simulink model "feedbackLineariz"  (Simulink 8.0)
settings: Solver=FixedStepDiscrete  StartTime=0.0  StopTime=inf  FixedStep=Ts  RelTol=1e-3
InitFcn:
  | initFeedLin;
values from neighbouring files (symbols this model uses):
  kp = diag([30*ones(1,3),7*ones(1,22)])    [initFeedLin.m]
libraries: WBCLibrary x11, utility x1
settings Model: Creator=iron  LastModifiedBy=daniele
settings DataIOCC: SignalLoggingSaveFormat=ModelDataLogs
settings DebuggingCC: FcnCallInpInsideContextMsg=UseLocalSettings
settings GRTTargetCC: CombineOutputUpdateFcns=off  GRTInterface=on

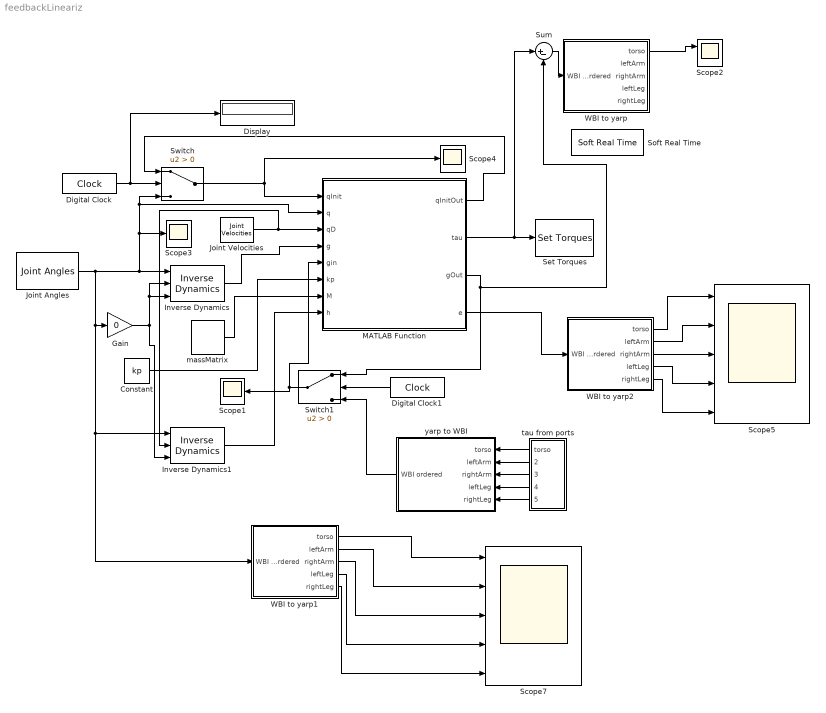
== system feedbackLineariz ==
  Constant : Constant  Value=kp
  Digital Clock : DigitalClock  SampleTime=-1
  Digital Clock1 : DigitalClock  SampleTime=-1
  Display : Display
  Gain : Gain  Gain=0
  Inverse Dynamics : WBCLibrary/wholeBodyModel/Dynamics/Inverse Dynamics  robotName=robotName  localName=localName
  Inverse Dynamics1 : WBCLibrary/wholeBodyModel/Dynamics/Inverse Dynamics  robotName=robotName  localName=localName
  Joint Angles : WBCLibrary/wholeBodyStates/Joint Angles  robotName=robotName  localName=localName
  Joint Velocities : WBCLibrary/wholeBodyStates/Joint Velocities  robotName=robotName  localName=localName
  MATLAB Function : MATLAB Function  TreatAsAtomicUnit=on
  Scope1 : Scope
      settings: YMin=-0.6  YMax=0.8
  Scope2 : Scope  NumInputPorts=2
      settings: YMin=-7~-5  YMax=6~5
  Scope3 : Scope
      settings: YMin=-0.6  YMax=0.8  SaveName=ScopeData3
  Scope4 : Scope
      settings: YMin=-0.6  YMax=0.8  SaveName=ScopeData4
  Scope5 : Scope  NumInputPorts=5
      settings: TimeRange=4.5  YMin=-0.1~-0.1~-0.2~-0.1~-0.1  YMax=0.3~0.3~0.2~0.3~0.3  SaveName=ScopeData2
  Scope7 : Scope  NumInputPorts=5
      settings: YMin=-0.5~-5~-5~-5~-5  YMax=4.75~5~5~5~5  SaveName=ScopeData6
  Set Torques : WBCLibrary/wholeBodyActuators/Set Torques  val=6  robotName=robotName  localName=localName
  Soft Real Time : utility/Soft Real Time  x=Ts
  Sum : Sum  Inputs=|+-
  Switch : Switch  Criteria=u2 > Threshold
  Switch1 : Switch  Criteria=u2 > Threshold
  WBI to yarp : Subsystem
  WBI to yarp1 : Subsystem
  WBI to yarp2 : Subsystem
  massMatrix : WBCLibrary/wholeBodyModel/Dynamics/massMatrix  val=8  robotname=robotName  localname=localName
  tau from ports : Subsystem
  yarp to WBI : Subsystem
  wires:
  Joint Angles/1 -> Inverse Dynamics1/1, WBI to yarp1/1(WBI ordered), Gain/1, Scope3/1, MATLAB Function/2(q), Switch/3, Inverse Dynamics/1
  Gain/1 -> Inverse Dynamics/2, Inverse Dynamics/3, Inverse Dynamics1/3
  Digital Clock/1 -> Display/1, Switch/2
  Switch/1 -> Scope4/1, MATLAB Function/1(qInit)
  MATLAB Function/1(qInitOut) -> Switch/1
  Joint Velocities/1 -> Inverse Dynamics1/2, MATLAB Function/3(qD)
  MATLAB Function/2(tau) -> Sum/1, Set Torques/1
  Digital Clock1/1 -> Switch1/2
  tau from ports/1(torso) -> yarp to WBI/1(torso)
  tau from ports/2(leftArm) -> yarp to WBI/2(leftArm)
  tau from ports/3(rightArm) -> yarp to WBI/3(rightArm)
  tau from ports/4(leftLeg) -> yarp to WBI/4(leftLeg)
  tau from ports/5(rightLeg) -> yarp to WBI/5(rightLeg)
  Switch1/1 -> Scope1/1, MATLAB Function/5(gin)
  MATLAB Function/3(gOut) -> Sum/2, Switch1/1
  yarp to WBI/1(WBI ordered) -> Switch1/3
  Constant/1 -> MATLAB Function/6(kp)
  Inverse Dynamics/1 -> MATLAB Function/4(g)
  massMatrix/1 -> MATLAB Function/7(M)
  Inverse Dynamics1/1 -> MATLAB Function/8(h)
  WBI to yarp/1(torso) -> Scope2/1
  Sum/1 -> WBI to yarp/1(WBI ordered)
  WBI to yarp1/1(torso) -> Scope7/1
  WBI to yarp1/2(leftArm) -> Scope7/2
  WBI to yarp1/3(rightArm) -> Scope7/3
  WBI to yarp1/4(leftLeg) -> Scope7/4
  WBI to yarp1/5(rightLeg) -> Scope7/5
  WBI to yarp2/2(leftArm) -> Scope5/2
  WBI to yarp2/1(torso) -> Scope5/1
  WBI to yarp2/3(rightArm) -> Scope5/3
  WBI to yarp2/4(leftLeg) -> Scope5/4
  WBI to yarp2/5(rightLeg) -> Scope5/5
  MATLAB Function/4(e) -> WBI to yarp2/1(WBI ordered)

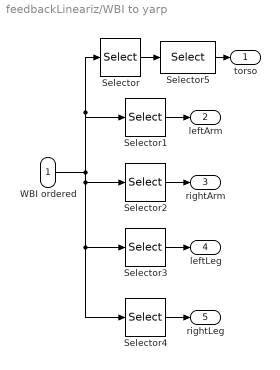
== system feedbackLineariz/WBI to yarp ==
  WBI ordered : Inport
  Selector : Selector  InputPortWidth=25  IndexOptions=Index vector (dialog)  Indices=[1 2 3]  OutputSizes=1
  Selector1 : Selector  InputPortWidth=25  IndexOptions=Index vector (dialog)  Indices=[4 5 6 7 8]  OutputSizes=1
  Selector2 : Selector  InputPortWidth=25  IndexOptions=Index vector (dialog)  Indices=[9 10 11 12 13]  OutputSizes=1
  Selector3 : Selector  InputPortWidth=25  IndexOptions=Index vector (dialog)  Indices=[14 15 16 17 18 19]  OutputSizes=1
  Selector4 : Selector  InputPortWidth=25  IndexOptions=Index vector (dialog)  Indices=[20 21 22 23 24 25]  OutputSizes=1
  Selector5 : Selector  InputPortWidth=3  IndexOptions=Index vector (dialog)  Indices=[3 2 1]  OutputSizes=1
  torso : Outport
  leftArm : Outport  Port=2
  rightArm : Outport  Port=3
  leftLeg : Outport  Port=4
  rightLeg : Outport  Port=5
  wires:
  Selector1/1 -> leftArm/1
  Selector2/1 -> rightArm/1
  Selector3/1 -> leftLeg/1
  Selector4/1 -> rightLeg/1
  WBI ordered/1 -> Selector/1, Selector1/1, Selector2/1, Selector4/1, Selector3/1
  Selector/1 -> Selector5/1
  Selector5/1 -> torso/1

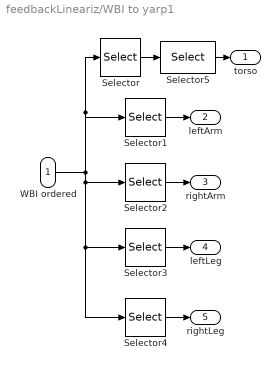
== system feedbackLineariz/WBI to yarp1 ==
  WBI ordered : Inport
  Selector : Selector  InputPortWidth=25  IndexOptions=Index vector (dialog)  Indices=[1 2 3]  OutputSizes=1
  Selector1 : Selector  InputPortWidth=25  IndexOptions=Index vector (dialog)  Indices=[4 5 6 7 8]  OutputSizes=1
  Selector2 : Selector  InputPortWidth=25  IndexOptions=Index vector (dialog)  Indices=[9 10 11 12 13]  OutputSizes=1
  Selector3 : Selector  InputPortWidth=25  IndexOptions=Index vector (dialog)  Indices=[14 15 16 17 18 19]  OutputSizes=1
  Selector4 : Selector  InputPortWidth=25  IndexOptions=Index vector (dialog)  Indices=[20 21 22 23 24 25]  OutputSizes=1
  Selector5 : Selector  InputPortWidth=3  IndexOptions=Index vector (dialog)  Indices=[3 2 1]  OutputSizes=1
  torso : Outport
  leftArm : Outport  Port=2
  rightArm : Outport  Port=3
  leftLeg : Outport  Port=4
  rightLeg : Outport  Port=5
  wires:
  Selector1/1 -> leftArm/1
  Selector2/1 -> rightArm/1
  Selector3/1 -> leftLeg/1
  Selector4/1 -> rightLeg/1
  WBI ordered/1 -> Selector/1, Selector1/1, Selector2/1, Selector4/1, Selector3/1
  Selector/1 -> Selector5/1
  Selector5/1 -> torso/1

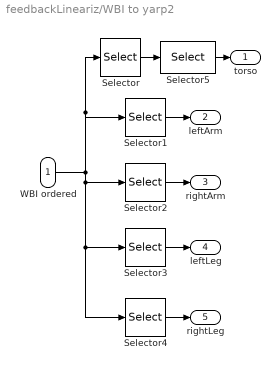
== system feedbackLineariz/WBI to yarp2 ==
  WBI ordered : Inport
  Selector : Selector  InputPortWidth=25  IndexOptions=Index vector (dialog)  Indices=[1 2 3]  OutputSizes=1
  Selector1 : Selector  InputPortWidth=25  IndexOptions=Index vector (dialog)  Indices=[4 5 6 7 8]  OutputSizes=1
  Selector2 : Selector  InputPortWidth=25  IndexOptions=Index vector (dialog)  Indices=[9 10 11 12 13]  OutputSizes=1
  Selector3 : Selector  InputPortWidth=25  IndexOptions=Index vector (dialog)  Indices=[14 15 16 17 18 19]  OutputSizes=1
  Selector4 : Selector  InputPortWidth=25  IndexOptions=Index vector (dialog)  Indices=[20 21 22 23 24 25]  OutputSizes=1
  Selector5 : Selector  InputPortWidth=3  IndexOptions=Index vector (dialog)  Indices=[3 2 1]  OutputSizes=1
  torso : Outport
  leftArm : Outport  Port=2
  rightArm : Outport  Port=3
  leftLeg : Outport  Port=4
  rightLeg : Outport  Port=5
  wires:
  Selector1/1 -> leftArm/1
  Selector2/1 -> rightArm/1
  Selector3/1 -> leftLeg/1
  Selector4/1 -> rightLeg/1
  WBI ordered/1 -> Selector/1, Selector1/1, Selector2/1, Selector4/1, Selector3/1
  Selector/1 -> Selector5/1
  Selector5/1 -> torso/1

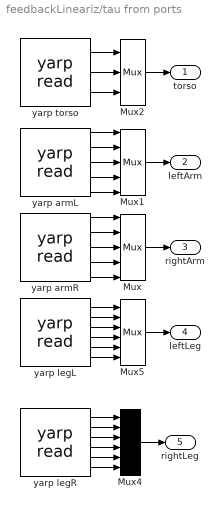
== system feedbackLineariz/tau from ports ==
  Mux : Mux  Inputs=5
  Mux1 : Mux  Inputs=5
  Mux2 : Mux  Inputs=3
  Mux4 : Mux  Inputs=6
  Mux5 : Mux  Inputs=6
  yarp armL : WBCLibrary/Utilities/yarp read  from='/icubGazeboSim/left_arm/analog:o/torques'  to='/tmp2:i'  num=5
  yarp armR : WBCLibrary/Utilities/yarp read  from='/icubGazeboSim/right_arm/analog:o/torques'  to='/tmp3:i'  num=5
  yarp legL : WBCLibrary/Utilities/yarp read  from='/icubGazeboSim/left_leg/analog:o/torques'  to='/tmp4:i'  num=6
  yarp legR : WBCLibrary/Utilities/yarp read  from='/icubGazeboSim/right_leg/analog:o/torques'  to='/tmp5:i'  num=6
  yarp torso : WBCLibrary/Utilities/yarp read  from='/icubGazeboSim/torso/analog:o/torques'  to='/tmp1:i'  num=3
  torso : Outport
  leftArm : Outport  Port=2
  rightArm : Outport  Port=3
  leftLeg : Outport  Port=4
  rightLeg : Outport  Port=5
  wires:
  yarp armR/1 -> Mux/1
  yarp armR/2 -> Mux/2
  yarp armR/3 -> Mux/3
  yarp armR/4 -> Mux/4
  yarp armR/5 -> Mux/5
  yarp armL/1 -> Mux1/1
  yarp armL/2 -> Mux1/2
  yarp armL/3 -> Mux1/3
  yarp armL/4 -> Mux1/4
  yarp armL/5 -> Mux1/5
  yarp torso/1 -> Mux2/1
  yarp torso/2 -> Mux2/2
  yarp torso/3 -> Mux2/3
  yarp legL/1 -> Mux5/1
  yarp legL/2 -> Mux5/2
  yarp legL/3 -> Mux5/3
  yarp legL/4 -> Mux5/4
  yarp legL/5 -> Mux5/5
  yarp legL/6 -> Mux5/6
  yarp legR/1 -> Mux4/1
  yarp legR/2 -> Mux4/2
  yarp legR/3 -> Mux4/3
  yarp legR/4 -> Mux4/4
  yarp legR/5 -> Mux4/5
  yarp legR/6 -> Mux4/6
  Mux2/1 -> torso/1
  Mux1/1 -> leftArm/1
  Mux/1 -> rightArm/1
  Mux5/1 -> leftLeg/1
  Mux4/1 -> rightLeg/1

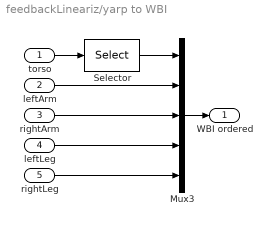
== system feedbackLineariz/yarp to WBI ==
  torso : Inport
  leftArm : Inport  Port=2
  rightArm : Inport  Port=3
  leftLeg : Inport  Port=4
  rightLeg : Inport  Port=5
  Mux3 : Mux  Inputs=5
  Selector : Selector  InputPortWidth=3  IndexOptions=Index vector (dialog)  Indices=[3 2 1]  OutputSizes=1
  WBI ordered : Outport
  wires:
  Selector/1 -> Mux3/1
  torso/1 -> Selector/1
  leftArm/1 -> Mux3/2
  rightArm/1 -> Mux3/3
  Mux3/1 -> WBI ordered/1
  leftLeg/1 -> Mux3/4
  rightLeg/1 -> Mux3/5

== matlab function MATLAB Function ==
  data: qInit input double; q input double; qInitOut output double; tau output double; qD input double; g input double; gin input double; gOut output double; kp input double; e output double; M input double; h input double
function [qInitOut,tau,gOut,e] = fcn(qInit,q,qD,g,gin,kp,M,h)
%#codegen

qInitOut = qInit;

kd = 0.3;

qDes = qInit-0.3;
% qDes(1) = qDes(1)+0.1;
% qDes(2) = qDes(2)-0.1;
e = (q-qDes);

gOut = gin;

% h = h(7:end);
M = M(7:end,7:end);


tau = h-(kp*e+kd.*qD);
% e = g - h;
% tau(3) = 0;
% tau(2) = 0;
% tau(1) = -14.6;
